simulink model "ohc_lowpass_filter"  (R2020b)
settings: Solver=FixedStepDiscrete  StartTime=0.0  StopTime=stopTime  FixedStep=2.0833333333333333e-05  RelTol=1e-3
values from neighbouring files (symbols this model uses):
  OHCLPcoeffs = [gainohc*c2LPohc gainohc*c2LPohc 0 1 -c1LPohc 0; gainohc*c2LPohc gainohc*c2LPohc 0 1 -c1LPohc 0]    [ohc_lowpass_filter_parameters.m]
settings Model: Creator=Ross  LastModifiedBy=conno
settings DataIOCC: SaveOutput=off  SaveTime=off  ReturnWorkspaceOutputs=off
settings OptimizationCC: BlockReduction=off  ConditionallyExecuteInputs=off  DefaultParameterBehavior=Inlined
settings DebuggingCC: ReadBeforeWriteMsg=DisableAll  WriteAfterWriteMsg=DisableAll  WriteAfterReadMsg=DisableAll  AlgebraicLoopMsg=error  MultiTaskDSMMsg=none  SingleTaskRateTransMsg=error  PregeneratedLibrarySubsystemCodeDiagnostic=none  ArithmeticOperatorsInVariantConditions=warning
settings HardwareCC: ProdBitPerPointer=32  ProdBitPerSizeT=32  ProdBitPerPtrDiffT=32  ProdLargestAtomicFloat=None  ProdIntDivRoundTo=Undefined  ProdEndianess=Unspecified  ProdWordSize=32  ProdHWDeviceType=ASIC/FPGA->ASIC/FPGA  TargetBitPerPointer=64  TargetBitPerSizeT=64  TargetBitPerPtrDiffT=64  TargetLongLongMode=on  TargetIntDivRoundTo=Zero  TargetEndianess=LittleEndian  TargetWordSize=64  TargetHWDeviceType=Custom Processor->MATLAB Host Computer  ProdEqTarget=off
settings ModelReferenceCC: UpdateModelReferenceTargets=IfOutOfDate
settings SFSimCC: SFSimEcho=off  SimUseLocalCustomCode=off  CustomCodeUndefinedFunction=UseInterfaceOnly
settings RTWCC: RTWUseLocalCustomCode=off

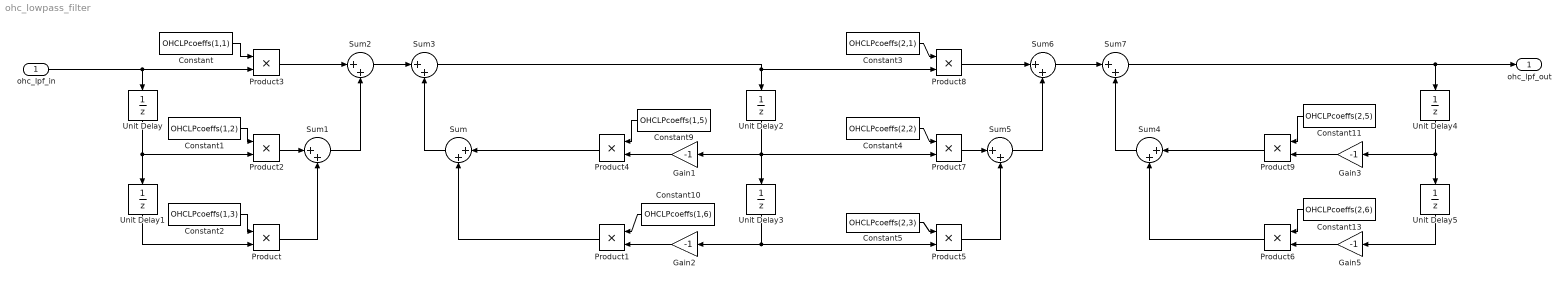
== system ohc_lowpass_filter ==
  ohc_lpf_in : Inport  OutDataTypeStr=single  PortDimensions=1  SampleTime=[2.0833333333333333e-05,0]
  Constant : Constant  Value=OHCLPcoeffs(1,1)  OutDataTypeStr=single  SampleTime=-1
  Constant1 : Constant  Value=OHCLPcoeffs(1,2)  OutDataTypeStr=single  SampleTime=-1
  Constant10 : Constant  Value=OHCLPcoeffs(1,6)  OutDataTypeStr=single  SampleTime=-1
  Constant11 : Constant  Value=OHCLPcoeffs(2,5)  OutDataTypeStr=single  SampleTime=-1
  Constant13 : Constant  Value=OHCLPcoeffs(2,6)  OutDataTypeStr=single  SampleTime=-1
  Constant2 : Constant  Value=OHCLPcoeffs(1,3)  OutDataTypeStr=single  SampleTime=-1
  Constant3 : Constant  Value=OHCLPcoeffs(2,1)  OutDataTypeStr=single  SampleTime=-1
  Constant4 : Constant  Value=OHCLPcoeffs(2,2)  OutDataTypeStr=single  SampleTime=-1
  Constant5 : Constant  Value=OHCLPcoeffs(2,3)  OutDataTypeStr=single  SampleTime=-1
  Constant9 : Constant  Value=OHCLPcoeffs(1,5)  OutDataTypeStr=single  SampleTime=-1
  Gain{1..3,5} (4 alike) : Gain  Gain=-1
  Product{,1..9} (10 alike) : Product
  Sum{,1..7} (8 alike) : Sum  Inputs=|++
  Unit Delay{,1..5} (6 alike) : UnitDelay  SampleTime=-1  HasFrameUpgradeWarning=on
  ohc_lpf_out : Outport  OutDataTypeStr=single  PortDimensions=1  SampleTime=[2.0833333333333333e-05,0]
  wires:
  Sum7/1 -> Unit Delay4/1, ohc_lpf_out/1
  Sum4/1 -> Sum7/2
  Sum3/1 -> Product8/2, Unit Delay2/1
  Sum/1 -> Sum3/2
  Product6/1 -> Sum4/2
  Product9/1 -> Sum4/1
  Product1/1 -> Sum/2
  Product4/1 -> Sum/1
  Sum6/1 -> Sum7/1
  Sum2/1 -> Sum3/1
  Product/1 -> Sum1/2
  Constant11/1 -> Product9/1
  Gain5/1 -> Product6/2
  Gain3/1 -> Product9/2
  Gain2/1 -> Product1/2
  Product8/1 -> Sum6/1
  Unit Delay5/1 -> Gain5/1
  Unit Delay1/1 -> Product/2
  Unit Delay3/1 -> Product5/2, Gain2/1
  Constant5/1 -> Product5/1
  Product5/1 -> Sum5/2
  Product2/1 -> Sum1/1
  Product3/1 -> Sum2/1
  Constant4/1 -> Product7/1
  Gain1/1 -> Product4/2
  Product7/1 -> Sum5/1
  Unit Delay4/1 -> Unit Delay5/1, Gain3/1
  Constant10/1 -> Product1/1
  Sum5/1 -> Sum6/2
  ohc_lpf_in/1 -> Product3/2, Unit Delay/1
  Unit Delay2/1 -> Product7/2, Unit Delay3/1, Gain1/1
  Constant9/1 -> Product4/1
  Constant1/1 -> Product2/1
  Constant/1 -> Product3/1
  Constant13/1 -> Product6/1
  Constant3/1 -> Product8/1
  Sum1/1 -> Sum2/2
  Unit Delay/1 -> Unit Delay1/1, Product2/2
  Constant2/1 -> Product/1
